simulink model "test"  (R2024b)
settings: Solver=VariableStepAuto  StartTime=0.0  StopTime=10.0  RelTol=1e-3
settings Model: Creator=Sagar  LastModifiedBy=Sagar

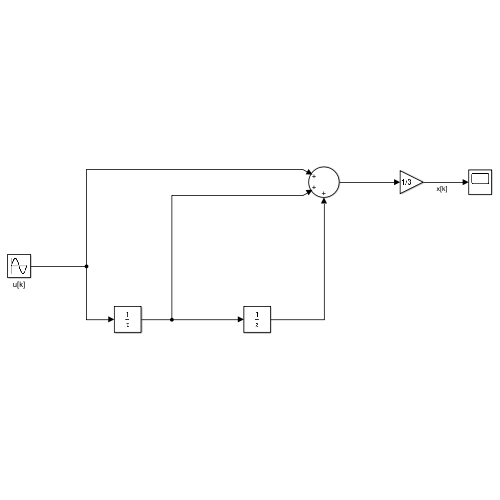
[thumbnail: Simulink's stored preview of the top-level diagram]
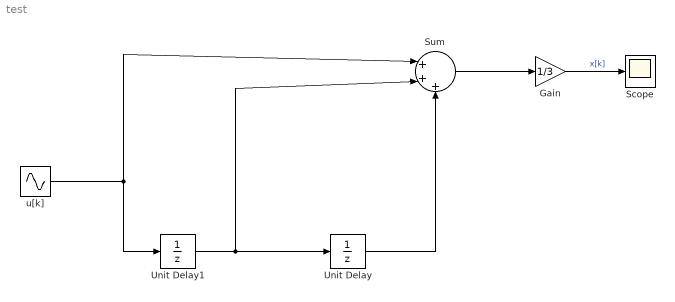
== system test ==
  Gain : Gain  Gain=1/3
  Scope : Scope
  Sum : Sum  Inputs=|+++
  Unit Delay : UnitDelay  SampleTime=-1  HasFrameUpgradeWarning=on
  Unit Delay1 : UnitDelay  SampleTime=-1  HasFrameUpgradeWarning=on
  u[k] : Sin  SampleTime=0
  wires:
  u[k]/1 -> Unit Delay1/1, Sum/1
  Unit Delay1/1 -> Sum/2, Unit Delay/1
  Unit Delay/1 -> Sum/3
  Sum/1 -> Gain/1
  Gain/1 -> Scope/1  "x[k]"
